simulink model "KR6_DirectKinematics"  (R2018a)
settings: Solver=VariableStepAuto  StartTime=0.0  StopTime=inf  RelTol=1e-3
libraries: vrlib x8, simulink x6, KR6_Lib x1
settings Model: Creator=Pedro Ramalho  LastModifiedBy=Pedro Ramalho

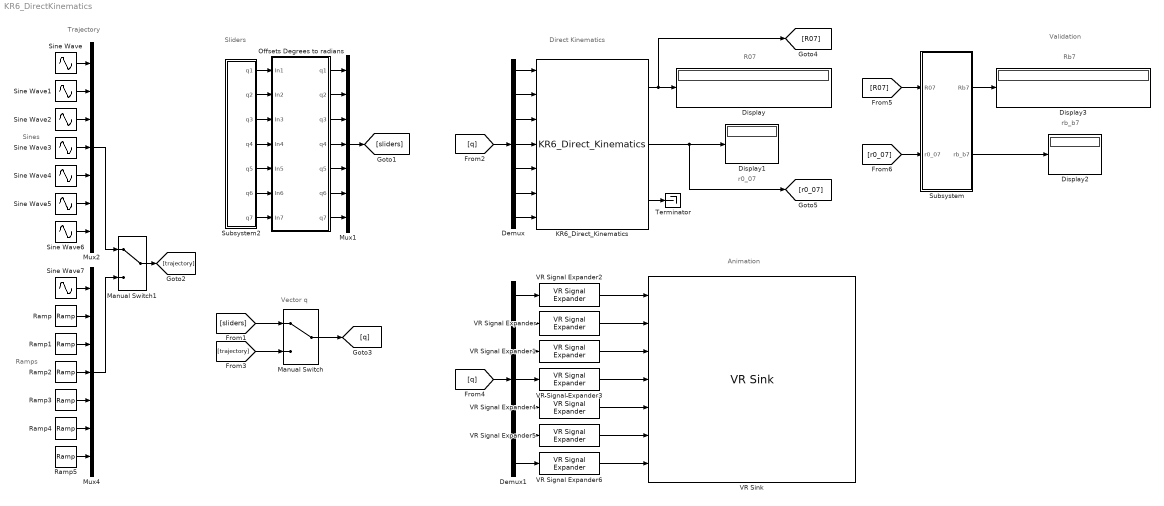
== system KR6_DirectKinematics ==
  note: Vector q
  note: Sliders
  note: Trajectory
  note: Animation
  note: Direct Kinematics
  note: R07
  note: r0_07
  note: Rb7
  note: rb_b7
  note: Sines
  note: Ramps
  note: Validation
  Demux : Demux  Outputs=7
  Demux1 : Demux  Outputs=7
  Display{,1..3} (4 alike) : Display
      Display settings: Decimation=2
  KR6_Direct_Kinematics : KR6_Lib/KR6_Direct_Kinematics
  Manual Switch : ManualSwitch
  Manual Switch1 : ManualSwitch
  Mux1 : Mux  Inputs=7
  Mux2 : Mux  Inputs=7
  Mux4 : Mux  Inputs=7
  Offsets Degrees to radians : Subsystem
  Ramp : simulink/Sources/Ramp  slope=0.5  start=0  InitialOutput=0
  Ramp1 : simulink/Sources/Ramp  slope=0  start=0  InitialOutput=-pi/2
  Ramp2 : simulink/Sources/Ramp  slope=0  start=0  InitialOutput=0
  Ramp3 : simulink/Sources/Ramp  slope=0  start=0  InitialOutput=0
  Ramp4 : simulink/Sources/Ramp  slope=0  start=0  InitialOutput=0
  Ramp5 : simulink/Sources/Ramp  slope=0  start=0  InitialOutput=-pi
  Sine Wave : Sin  Frequency=0.2  SampleTime=0
  Sine Wave1 : Sin  Amplitude=3  Frequency=0.2  SampleTime=0
  Sine Wave2 : Sin  Bias=-1.5  Frequency=0.2  SampleTime=0
  Sine Wave3 : Sin  Amplitude=0.5  Frequency=0.2  SampleTime=0
  Sine Wave4 : Sin  Frequency=0.2  SampleTime=0
  Sine Wave5 : Sin  Amplitude=1.5  Frequency=0.2  SampleTime=0
  Sine Wave6 : Sin  Amplitude=1.5  Frequency=0.2  SampleTime=0
  Sine Wave7 : Sin  Amplitude=0  Frequency=0.1  SampleTime=0
  Subsystem : Subsystem
  Subsystem2 : Subsystem  mask{q1=0.3, q2=45.01, q3=-45, q4=45, q5=45.07, q6=45.05, q7=45}
  Terminator : Terminator
  VR Signal Expander{,1,3..6} (6 alike) : vrlib/VR Signal Expander  outwidth=4  outidx=4
      settings: SourceProductName=Simulink 3D Animation  SourceProductBaseCode=VR
  VR Signal Expander2 : vrlib/VR Signal Expander  outwidth=3  outidx=3
      settings: SourceProductName=Simulink 3D Animation  SourceProductBaseCode=VR
  VR Sink : vrlib/VR Sink  InstantiateOnLoad=on  SampleTime=0.1  ViewEnable=on  RemoteChange=off  RemoteView=off  FieldsWritten=Jt1_DH_dv.translation.3.1.1.double#Jt2_DH_dv.rotation.4.1.1.double#Jt3_DH_dv.rotation.4.1.1.double#Jt4_DH_dv.rotation.4.1.1.double#Jt5_DH_dv.rotation.4.1.1.double#Jt6_DH_dv.rotation.4.1.1.double#Jt7_DH_dv.rotation.4.1.1.double  WorldFileName=vrrobotKR6.wrl  WorldDescription=D-H Reference Frames for Virtual Reality Robot  AutoView=off  VideoDimensions=[]  AllowVariableSize=off
      settings: SourceProductBaseCode=VR
  wires:
  KR6_Direct_Kinematics/1 -> Display/1, [R07]
  KR6_Direct_Kinematics/2 -> Display1/1, [r0_07]
  VR Signal Expander2/1 -> VR Sink/1
  VR Signal Expander/1 -> VR Sink/2
  VR Signal Expander1/1 -> VR Sink/3
  VR Signal Expander3/1 -> VR Sink/4
  VR Signal Expander4/1 -> VR Sink/5
  VR Signal Expander5/1 -> VR Sink/6
  VR Signal Expander6/1 -> VR Sink/7
  KR6_Direct_Kinematics/3 -> Terminator/1
  Sine Wave/1 -> Mux2/1
  Subsystem2/1(q1) -> Offsets Degrees to radians/1(In1)
  Subsystem2/2(q2) -> Offsets Degrees to radians/2(In2)
  Subsystem2/3(q3) -> Offsets Degrees to radians/3(In3)
  Subsystem2/4(q4) -> Offsets Degrees to radians/4(In4)
  Subsystem2/5(q5) -> Offsets Degrees to radians/5(In5)
  Subsystem2/6(q6) -> Offsets Degrees to radians/6(In6)
  Subsystem2/7(q7) -> Offsets Degrees to radians/7(In7)
  Offsets Degrees to radians/1(q1) -> Mux1/1
  Offsets Degrees to radians/2(q2) -> Mux1/2
  Offsets Degrees to radians/3(q3) -> Mux1/3
  Offsets Degrees to radians/4(q4) -> Mux1/4
  Offsets Degrees to radians/5(q5) -> Mux1/5
  Offsets Degrees to radians/6(q6) -> Mux1/6
  Offsets Degrees to radians/7(q7) -> Mux1/7
  [sliders] -> Manual Switch/1
  [trajectory] -> Manual Switch/2
  Mux1/1 -> [sliders]
  Demux/1 -> KR6_Direct_Kinematics/1
  Demux/2 -> KR6_Direct_Kinematics/2
  Demux/3 -> KR6_Direct_Kinematics/3
  Demux/4 -> KR6_Direct_Kinematics/4
  Demux/5 -> KR6_Direct_Kinematics/5
  Demux/6 -> KR6_Direct_Kinematics/6
  Demux/7 -> KR6_Direct_Kinematics/7
  [q] -> Demux/1
  [q] -> Demux1/1
  Demux1/1 -> VR Signal Expander2/1
  Demux1/3 -> VR Signal Expander1/1
  Demux1/6 -> VR Signal Expander5/1
  Demux1/2 -> VR Signal Expander/1
  Demux1/5 -> VR Signal Expander4/1
  Demux1/4 -> VR Signal Expander3/1
  Demux1/7 -> VR Signal Expander6/1
  Manual Switch/1 -> [q]
  Sine Wave1/1 -> Mux2/2
  Sine Wave2/1 -> Mux2/3
  Sine Wave3/1 -> Mux2/4
  Sine Wave4/1 -> Mux2/5
  Sine Wave5/1 -> Mux2/6
  Sine Wave6/1 -> Mux2/7
  Mux2/1 -> Manual Switch1/1
  Manual Switch1/1 -> [trajectory]
  Ramp/1 -> Mux4/2
  Ramp1/1 -> Mux4/3
  Ramp2/1 -> Mux4/4
  Ramp4/1 -> Mux4/6
  Ramp5/1 -> Mux4/7
  Sine Wave7/1 -> Mux4/1
  Mux4/1 -> Manual Switch1/2
  Ramp3/1 -> Mux4/5
  Subsystem/2(rb_b7) -> Display2/1
  [R07] -> Subsystem/1(R07)
  [r0_07] -> Subsystem/2(r0_07)
  Subsystem/1(Rb7) -> Display3/1

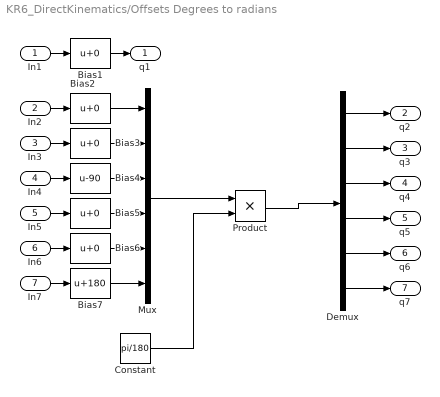
== system KR6_DirectKinematics/Offsets Degrees to radians ==
  In1 : Inport
  In2 : Inport  Port=2
  In3 : Inport  Port=3
  In4 : Inport  Port=4
  In5 : Inport  Port=5
  In6 : Inport  Port=6
  In7 : Inport  Port=7
  Bias{1..3,5..6} (5 alike) : Bias
  Bias4 : Bias  Bias=-90
  Bias7 : Bias  Bias=180
  Constant : Constant  Value=pi/180
  Demux : Demux  Outputs=6
  Mux : Mux  Inputs=6
  Product : Product
  q1 : Outport
  q2 : Outport  Port=2
  q3 : Outport  Port=3
  q4 : Outport  Port=4
  q5 : Outport  Port=5
  q6 : Outport  Port=6
  q7 : Outport  Port=7
  wires:
  In6/1 -> Bias6/1
  In5/1 -> Bias5/1
  In3/1 -> Bias3/1
  In1/1 -> Bias1/1
  Bias1/1 -> q1/1
  In7/1 -> Bias7/1
  In4/1 -> Bias4/1
  In2/1 -> Bias2/1
  Bias7/1 -> Mux/6
  Bias2/1 -> Mux/1
  Bias3/1 -> Mux/2
  Bias4/1 -> Mux/3
  Bias5/1 -> Mux/4
  Bias6/1 -> Mux/5
  Mux/1 -> Product/1
  Constant/1 -> Product/2
  Demux/1 -> q2/1
  Demux/2 -> q3/1
  Demux/3 -> q4/1
  Demux/4 -> q5/1
  Demux/5 -> q6/1
  Demux/6 -> q7/1
  Product/1 -> Demux/1

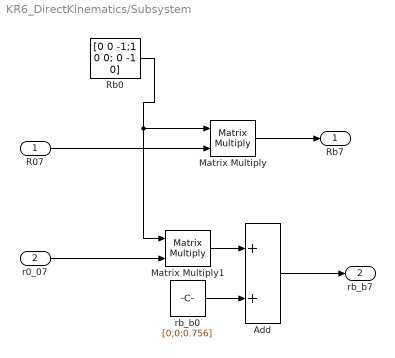
== system KR6_DirectKinematics/Subsystem ==
  R07 : Inport
  r0_07 : Inport  Port=2
  Add : Sum
  Matrix Multiply : Product  Multiplication=Matrix(*)
  Matrix Multiply1 : Product  Multiplication=Matrix(*)
  Rb0 : Constant  Value=[0 0 -1;1 0 0; 0 -1 0]
  rb_b0 : Constant  Value=[0;0;0.756]
  Rb7 : Outport
  rb_b7 : Outport  Port=2
  wires:
  R07/1 -> Matrix Multiply/2
  r0_07/1 -> Matrix Multiply1/2
  Matrix Multiply/1 -> Rb7/1
  Rb0/1 -> Matrix Multiply1/1, Matrix Multiply/1
  Matrix Multiply1/1 -> Add/1
  rb_b0/1 -> Add/2
  Add/1 -> rb_b7/1

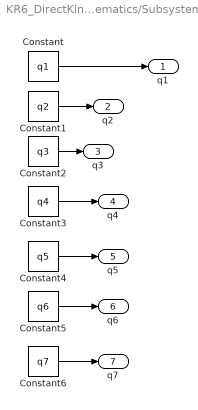
== system KR6_DirectKinematics/Subsystem2 ==
  Constant : Constant  Value=q1
  Constant1 : Constant  Value=q2
  Constant2 : Constant  Value=q3
  Constant3 : Constant  Value=q4
  Constant4 : Constant  Value=q5
  Constant5 : Constant  Value=q6
  Constant6 : Constant  Value=q7
  q1 : Outport
  q2 : Outport  Port=2
  q3 : Outport  Port=3
  q4 : Outport  Port=4
  q5 : Outport  Port=5
  q6 : Outport  Port=6
  q7 : Outport  Port=7
  wires:
  Constant/1 -> q1/1
  Constant2/1 -> q3/1
  Constant1/1 -> q2/1
  Constant3/1 -> q4/1
  Constant4/1 -> q5/1
  Constant5/1 -> q6/1
  Constant6/1 -> q7/1
